simulink model "COMPONENT_model_MEME"  (R2019a)
settings: Solver=ode45  StartTime=0.0  StopTime=60  FixedStep=0.001  RelTol=1e-6  EnableMultiTasking=on
undefined symbols (not defined in the file): d, Ic_xx_val, Io, m, pm_0
settings Model: Creator=bhorton  LastModifiedBy=bhorton
settings SolverCC: ZeroCrossAlgorithm=Adaptive
settings DataIOCC: SaveOutput=off  SignalLogging=off  DSMLogging=off  VisualizeSimOutput=off  SaveTime=off  ReturnWorkspaceOutputs=off
settings OptimizationCC: LifeSpan=inf
settings DebuggingCC: AllowSymbolicDim=off  SFUnexpectedBacktrackingDiag=warning  SFNoUnconditionalDefaultTransitionDiag=warning  SFExecutionAtInitializationDiag=none  ArithmeticOperatorsInVariantConditions=warning
settings ModelReferenceCC: PropagateSignalLabelsOutOfModel=off
settings SFSimCC: SimUseLocalCustomCode=off
settings RTWCC: RTWUseLocalCustomCode=off
settings CodeAppCC: StateflowObjectComments=on
settings GRTTargetCC: TargetLangStandard=C89/C90 (ANSI)
settings ConfigComp: CovMetricSettings=dw  CovHtmlReporting=on  CovSaveCumulativeToWorkspaceVar=on  CovSaveSingleToWorkspaceVar=on  CovExternalEMLEnable=off
settings SimscapeCC: SimscapeNormalizeSystem=off

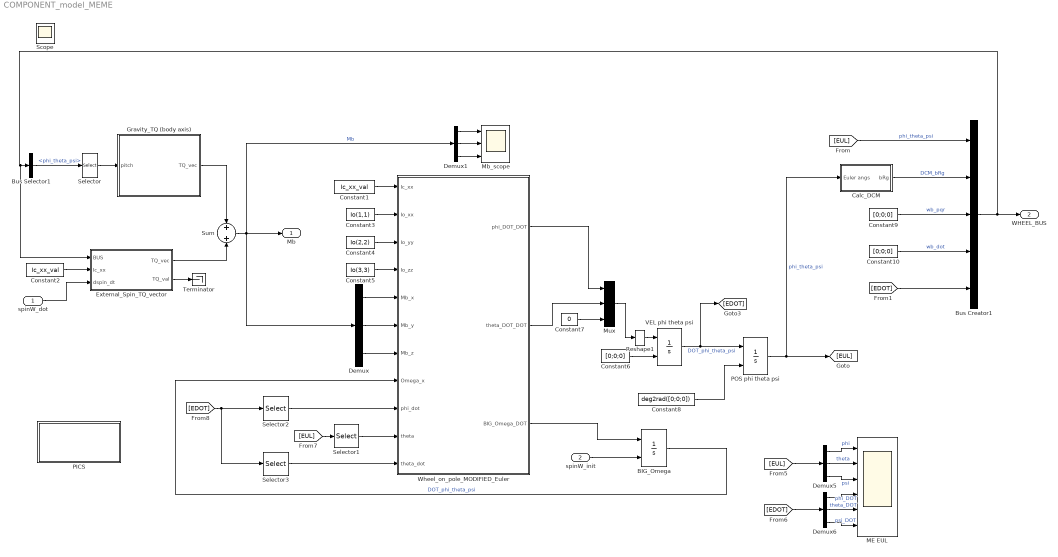
== system COMPONENT_model_MEME ==
  spinW_dot : Inport
  spinW_init : Inport  Port=2
  BIG_Omega : Integrator  InitialConditionSource=external  InitialCondition=pm_0
  Bus Creator1 : BusCreator  Inputs=5
  Bus Selector1 : BusSelector  OutputSignals=phi_theta_psi
  Calc_DCM : Subsystem
  Constant1 : Constant  Value=Ic_xx_val
  Constant10 : Constant  Value=[0;0;0]  VectorParams1D=off
  Constant2 : Constant  Value=Ic_xx_val
  Constant3 : Constant  Value=Io(1,1)
  Constant4 : Constant  Value=Io(2,2)
  Constant5 : Constant  Value=Io(3,3)
  Constant6 : Constant  Value=[0;0;0]  VectorParams1D=off
  Constant7 : Constant  Value=0  VectorParams1D=off
  Constant8 : Constant  Value=deg2rad([0;0;0])  VectorParams1D=off
  Constant9 : Constant  Value=[0;0;0]  VectorParams1D=off
  Demux{,1,5..6} (4 alike) : Demux  Outputs=3
  External_Spin_TQ_vector : Subsystem
  Gravity_TQ (body axis) : Subsystem
  ME EUL : Scope  NumInputPorts=6
  Mb_scope : Scope  NumInputPorts=3
  Mux : Mux  Inputs=3
  PICS : Subsystem
  POS phi theta psi : Integrator  InitialConditionSource=external  InitialCondition=pm_0
  Reshape1 : Reshape  OutputDimensionality=Column vector (2-D)
  Selector : Selector  InputPortWidth=3  IndexOptions=Index vector (dialog)  Indices=2  OutputSizes=1
  Selector1 : Selector  InputPortWidth=3  IndexOptions=Index vector (dialog)  Indices=2  OutputSizes=1
  Selector2 : Selector  InputPortWidth=3  IndexOptions=Index vector (dialog)  Indices=1  OutputSizes=1
  Selector3 : Selector  InputPortWidth=3  IndexOptions=Index vector (dialog)  Indices=2  OutputSizes=1
  Sum : Sum  Inputs=+|+
  Terminator : Terminator
  VEL phi theta psi : Integrator  InitialConditionSource=external  InitialCondition=pm_0
  Wheel_on_pole_MODIFIED_Euler : MATLAB Function  TreatAsAtomicUnit=on
  Mb : Outport
  WHEEL_BUS : Outport  Port=2  OutDataTypeStr=Bus: EME_BUS
  Scope : Scope
  wires:
  Mux/1 -> Reshape1/1
  Gravity_TQ (body axis)/1(TQ_vec) -> Sum/1
  Selector/1 -> Gravity_TQ (body axis)/1(pitch)
  POS phi theta psi/1 -> Calc_DCM/1(Euler angs), [EUL]  "phi_theta_psi"
  [EUL] -> Selector1/1
  [EDOT] -> Selector3/1, Selector2/1
  Demux1/1 -> Mb_scope/1
  Sum/1 -> Demux1/1, Demux/1, Mb/1  "Mb"
  VEL phi theta psi/1 -> POS phi theta psi/1, [EDOT]  "DOT_phi_theta_psi"
  Demux6/1 -> ME EUL/4  "phi_DOT"
  Demux6/3 -> ME EUL/6  "psi_DOT"
  BIG_Omega/1 -> Wheel_on_pole_MODIFIED_Euler/8(Omega_x)  "DOT_phi_theta_psi"
  Calc_DCM/1(bRg) -> Bus Creator1/2  "DCM_bRg"
  Demux1/3 -> Mb_scope/3
  External_Spin_TQ_vector/1(TQ_vec) -> Sum/2
  Wheel_on_pole_MODIFIED_Euler/1(phi_DOT_DOT) -> Mux/1
  Wheel_on_pole_MODIFIED_Euler/3(BIG_Omega_DOT) -> BIG_Omega/1
  Constant5/1 -> Wheel_on_pole_MODIFIED_Euler/4(Io_zz)
  Wheel_on_pole_MODIFIED_Euler/2(theta_DOT_DOT) -> Mux/2
  Constant2/1 -> External_Spin_TQ_vector/2(Ic_xx)
  [EDOT] -> Demux6/1
  Demux5/2 -> ME EUL/2  "theta"
  Selector1/1 -> Wheel_on_pole_MODIFIED_Euler/10(theta)
  Constant3/1 -> Wheel_on_pole_MODIFIED_Euler/2(Io_xx)
  Demux/3 -> Wheel_on_pole_MODIFIED_Euler/7(Mb_z)
  Constant1/1 -> Wheel_on_pole_MODIFIED_Euler/1(Ic_xx)
  Constant7/1 -> Mux/3
  spinW_dot/1 -> External_Spin_TQ_vector/3(dspin_dt)
  [EUL] -> Demux5/1
  Selector2/1 -> Wheel_on_pole_MODIFIED_Euler/9(phi_dot)
  External_Spin_TQ_vector/2(TQ_val) -> Terminator/1
  Reshape1/1 -> VEL phi theta psi/1
  Constant8/1 -> POS phi theta psi/2
  spinW_init/1 -> BIG_Omega/2
  Demux6/2 -> ME EUL/5  "theta_DOT"
  Constant6/1 -> VEL phi theta psi/2
  Demux1/2 -> Mb_scope/2
  Demux5/1 -> ME EUL/1  "phi"
  Demux5/3 -> ME EUL/3  "psi"
  Demux/2 -> Wheel_on_pole_MODIFIED_Euler/6(Mb_y)
  Bus Selector1/1 -> Selector/1  "<phi_theta_psi>"
  Demux/1 -> Wheel_on_pole_MODIFIED_Euler/5(Mb_x)
  Selector3/1 -> Wheel_on_pole_MODIFIED_Euler/11(theta_dot)
  Constant4/1 -> Wheel_on_pole_MODIFIED_Euler/3(Io_yy)
  Constant10/1 -> Bus Creator1/4  "wb_dot"
  [EUL] -> Bus Creator1/1  "phi_theta_psi"
  Constant9/1 -> Bus Creator1/3  "wb_pqr"
  [EDOT] -> Bus Creator1/5
  Bus Creator1/1 -> External_Spin_TQ_vector/1(BUS), Bus Selector1/1, WHEEL_BUS/1

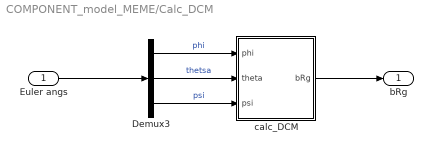
== system COMPONENT_model_MEME/Calc_DCM ==
  Euler angs : Inport
  Demux3 : Demux  Outputs=3
  calc_DCM : MATLAB Function  TreatAsAtomicUnit=on
  bRg : Outport
  wires:
  calc_DCM/1(bRg) -> bRg/1
  Demux3/3 -> calc_DCM/3(psi)  "psi"
  Demux3/2 -> calc_DCM/2(theta)  "thetsa"
  Demux3/1 -> calc_DCM/1(phi)  "phi"
  Euler angs/1 -> Demux3/1

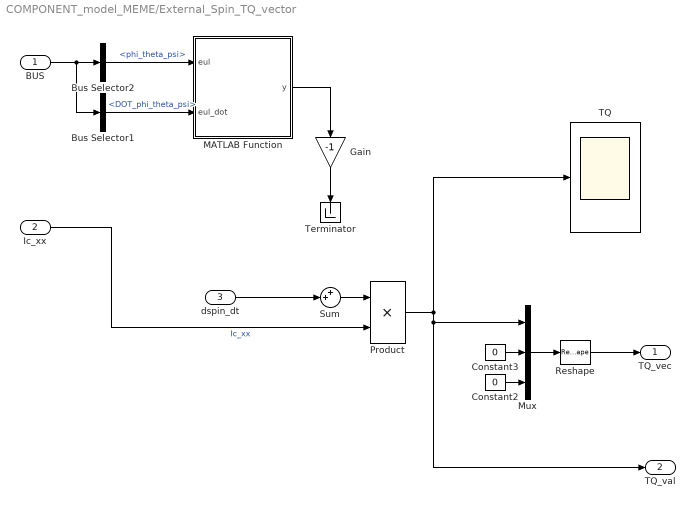
== system COMPONENT_model_MEME/External_Spin_TQ_vector ==
  BUS : Inport
  Ic_xx : Inport  Port=2
  dspin_dt : Inport  Port=3
  Bus Selector1 : BusSelector  OutputSignals=DOT_phi_theta_psi
  Bus Selector2 : BusSelector  OutputSignals=phi_theta_psi
  Constant2 : Constant  Value=0
  Constant3 : Constant  Value=0
  Gain : Gain  Gain=-1
  MATLAB Function : MATLAB Function  TreatAsAtomicUnit=on
  Mux : Mux  Inputs=3
  Product : Product
  Reshape : Reshape  OutputDimensionality=Column vector (2-D)
  Sum : Sum  Inputs=++|
  TQ : Scope
  Terminator : Terminator
  TQ_vec : Outport
  TQ_val : Outport  Port=2
  wires:
  Mux/1 -> Reshape/1
  Reshape/1 -> TQ_vec/1
  Product/1 -> TQ/1, TQ_val/1, Mux/1
  Constant2/1 -> Mux/3
  Ic_xx/1 -> Product/2  "Ic_xx"
  Constant3/1 -> Mux/2
  BUS/1 -> Bus Selector1/1, Bus Selector2/1
  Bus Selector2/1 -> MATLAB Function/1(eul)  "<phi_theta_psi>"
  Bus Selector1/1 -> MATLAB Function/2(eul_dot)  "<DOT_phi_theta_psi>"
  dspin_dt/1 -> Sum/2
  MATLAB Function/1(y) -> Gain/1
  Gain/1 -> Terminator/1
  Sum/1 -> Product/1

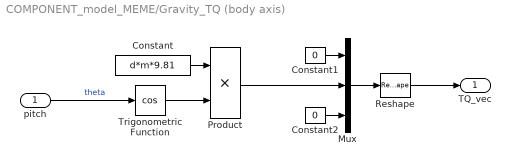
== system COMPONENT_model_MEME/Gravity_TQ (body axis) ==
  pitch : Inport
  Constant : Constant  Value=d*m*9.81
  Constant1 : Constant  Value=0
  Constant2 : Constant  Value=0
  Mux : Mux  Inputs=3
  Product : Product
  Reshape : Reshape  OutputDimensionality=Column vector (2-D)
  Trigonometric Function : Trigonometry  Operator=cos
  TQ_vec : Outport
  wires:
  Mux/1 -> Reshape/1
  Reshape/1 -> TQ_vec/1
  Trigonometric Function/1 -> Product/2
  pitch/1 -> Trigonometric Function/1  "theta"
  Constant/1 -> Product/1
  Constant1/1 -> Mux/1
  Product/1 -> Mux/2
  Constant2/1 -> Mux/3

== system COMPONENT_model_MEME/PICS ==

== matlab function COMPONENT_model_MEME/Wheel_on_pole_MODIFIED_Euler ==
  data: Ic_xx input; phi_DOT_DOT output; Io_xx input; Io_yy input; Io_zz input; Mb_x input; Mb_y input; Mb_z input; Omega_x input; phi_dot input; theta input; theta_dot input; theta_DOT_DOT output; BIG_Omega_DOT output
function [phi_DOT_DOT,theta_DOT_DOT,BIG_Omega_DOT] = tmp_block(Ic_xx,Io_xx,Io_yy,Io_zz,Mb_x,Mb_y,Mb_z,Omega_x,phi_dot,theta,theta_dot)
%#codegen

%    This function was generated by the Symbolic Math Toolbox version 8.3.
%    19-Aug-2019 09:34:54

t2 = cos(theta);
t3 = sin(theta);
t4 = phi_dot.^2;
t7 = 1.0./Io_zz;
t5 = t2.^2;
t6 = t3.^2;
t8 = 1.0./t2;
phi_DOT_DOT = t7.*t8.*(Mb_z+Ic_xx.*Omega_x.*theta_dot-Io_xx.*phi_dot.*t3.*theta_dot+Io_yy.*phi_dot.*t3.*theta_dot+Io_zz.*phi_dot.*t3.*theta_dot);
if nargout > 1
    theta_DOT_DOT = (Mb_y+Io_xx.*t2.*t3.*t4-Io_zz.*t2.*t3.*t4-Ic_xx.*Omega_x.*phi_dot.*t2)./Io_yy;
end
if nargout > 2
    BIG_Omega_DOT = (t7.*t8.*(Io_xx.*Mb_z.*t3+Io_zz.*Mb_x.*t2-Io_xx.^2.*phi_dot.*t6.*theta_dot-phi_dot.*t5.*1.0./t7.^2.*theta_dot+Ic_xx.*Io_xx.*Omega_x.*t3.*theta_dot+Io_xx.*Io_yy.*phi_dot.*t6.*theta_dot+Io_xx.*Io_zz.*phi_dot.*t5.*theta_dot+Io_xx.*Io_zz.*phi_dot.*t6.*theta_dot+Io_yy.*Io_zz.*phi_dot.*t5.*theta_dot))./Ic_xx;
end

== matlab function COMPONENT_model_MEME/External_Spin_TQ_vector/MATLAB Function ==
  data: eul input; y output; eul_dot input
function y = fcn(eul, eul_dot)

theta = eul(2);

phi_dot   = eul_dot(1); 
theta_dot = eul_dot(2);

y = phi_dot*theta_dot*cos(theta);

== matlab function COMPONENT_model_MEME/Calc_DCM/calc_DCM ==
  data: phi input; bRg output; theta input; psi input
function bRg = calc_bRg(phi, theta, psi)
%#codegen

bRg = [ ...
                              cos(phi)*cos(theta),                              cos(theta)*sin(phi),         -sin(theta);
 cos(phi)*sin(psi)*sin(theta) - cos(psi)*sin(phi), cos(phi)*cos(psi) + sin(phi)*sin(psi)*sin(theta), cos(theta)*sin(psi);
 sin(phi)*sin(psi) + cos(phi)*cos(psi)*sin(theta), cos(psi)*sin(phi)*sin(theta) - cos(phi)*sin(psi), cos(psi)*cos(theta);
 ];

end
